simulink model "evaporatortesting"  (R2018b)
settings: Solver=VariableStepAuto  StartTime=0.0  StopTime=20000  FixedStep=1e-8  RelTol=1e-3
settings Model: Creator=smf52  LastModifiedBy=art58

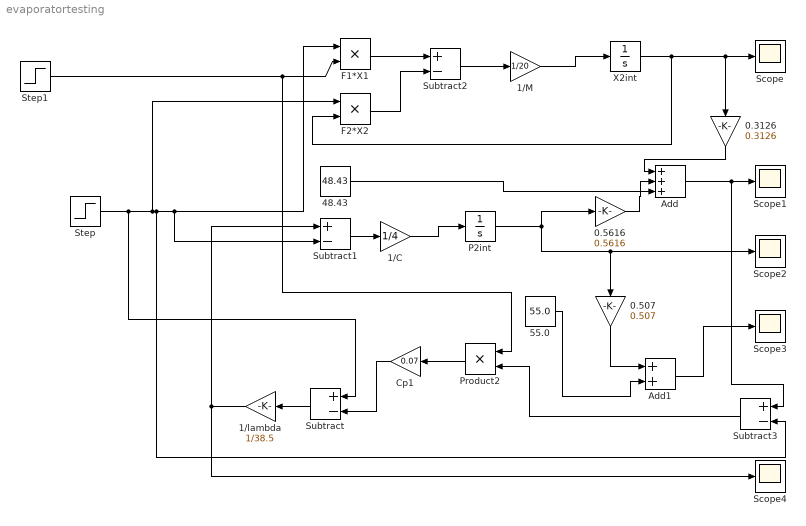
== system evaporatortesting ==
  0.3126 : Gain  Gain=0.3126
  0.507 : Gain  Gain=0.507
  0.5616 : Gain  Gain=0.5616
  1/C : Gain  Gain=1/4
  1/M : Gain  Gain=1/20
  1/lambda : Gain  Gain=1/38.5
  48.43 : Constant  Value=48.43
  55.0 : Constant  Value=55.0
  Add : Sum  Inputs=+++
  Add1 : Sum
  Cp1 : Gain  Gain=0.07
  F1*X1 : Product
  F2*X2 : Product
  P2int : Integrator
  Product2 : Product
  Scope{,1..4} (5 alike) : Scope
  Step : Step  SampleTime=0
  Step1 : Step  SampleTime=0
  Subtract{,1..3} (4 alike) : Sum  Inputs=+-
  X2int : Integrator
  wires:
  Subtract2/1 -> 1/M/1
  X2int/1 -> F2*X2/2, Scope/1, 0.3126/1
  Subtract1/1 -> 1/C/1
  1/C/1 -> P2int/1
  P2int/1 -> Scope2/1, 0.507/1, 0.5616/1
  Add/1 -> Scope1/1, Subtract3/1
  0.507/1 -> Add1/1
  Add1/1 -> Scope3/1
  0.5616/1 -> Add/2
  0.3126/1 -> Add/1
  48.43/1 -> Add/3
  55.0/1 -> Add1/2
  Step/1 -> Subtract3/2, Subtract1/2, F1*X1/1, F2*X2/1, Subtract/1
  Subtract3/1 -> Product2/2
  Product2/1 -> Cp1/1
  Subtract/1 -> 1/lambda/1
  1/lambda/1 -> Scope4/1, Subtract1/1
  F2*X2/1 -> Subtract2/2
  F1*X1/1 -> Subtract2/1
  1/M/1 -> X2int/1
  Step1/1 -> Product2/1, F1*X1/2
  Cp1/1 -> Subtract/2
